simulink model "pulse_generator_V"  (R2016b)
settings: Solver=FixedStepDiscrete  StartTime=0.0  StopTime=15  RelTol=1e-3
model workspace (MAT data in the model file):
  input_struct.time = [0; 1; 2; 3; 4; 5; 6; 7; 8; 9; 10; 11; 12; 13; 14; 15; 16; 17; 18; 19; 20; 21; 22; 23; 24; 25; 26; 27; 28; 29; 30; 31; 32; 33; 34; 35; 36; 37; 38; 39; 40; 41; 42; 43; 44; 45; 46; 47; 48; 49; 50; 51; 52; 53; 54; 55; 56; 57; 58; 59; 60; 61; 62; 63; 64; 65; 66; 67; 68; 69; 70; 71; 72; 73; 74; 75; 76; 77; 78; 79; 80; 81; 82; 83; 84; 85; 86; 87; 88; 89; 90; 91; 92; 93; 94; 95; 96; 97; 98; 99; 100]
  input_struct.signals.name = 'In1'
  input_struct.signals.values = [79.4284540684; 31.1215042045; 52.8533135506; 16.56487295; 60.1981941402; 26.297128454; 65.4079098477; 68.921450314; 74.8151592824; 45.0541598502; 8.38213779969; 22.8976968717; 91.3337361502; 15.2378018969; 82.581697749; 53.834243526; 99.6134716627; 7.81755287532; 44.2678269775; 10.6652770181; 96.1898080855; 0.463422413407; 77.4910464712; 81.7303220653; 86.8694705364; 8.44358455109; 39.9782649099; 25.9870402851; 80.0068480224; 43.1413827464; 91.064759443; 18.1847028303; 26.3802916522; 14.5538980385; 13.6068558709; 86.929220764; 57.9704587366; 54.9860201836; 14.4954798224; 85.3031117722; 62.2055131485; 35.0952380892; 51.3249539867; 40.1808033752; 7.59666916908; 23.9916153554; 12.3318934835; 18.3907788282; 23.9952525665; 41.7267069084; 4.96544303257; 90.2716109915; 94.4787189722; 49.0864092468; 48.92526384; 33.7719409821; 90.0053846418; 36.924678112; 11.1202755294; 78.0252068321; 38.9738836961; 24.1691285914; 40.3912145588; 9.64545251684; 13.1973292606; 94.2050590775; 95.613454023; 57.5208595078; 5.97795429472; 23.4779913372; 35.3158571222; 82.1194040198; 1.54034376516; 4.30238016578; 16.8990029463; 64.9115474956; 73.1722385659; 64.7745963136; 45.0923706431; 54.7008892286; 29.6320805608; 74.4692807074; 18.8955015033; 68.6775433365; 18.3511155737; 36.848459649; 62.561856073; 78.0227435151; 8.11257688658; 92.9385970969; 77.5712678608; 48.6791632403; 43.5858588581; 44.678374943; 30.6349472017; 50.8508655381; 51.0771564172; 81.7627708322; 79.4831416883; 64.4318130194; 37.860938266]
  input_struct.signals.dimensions = 1
settings Model: Creator=hbourbou  LastModifiedBy=hbourbou

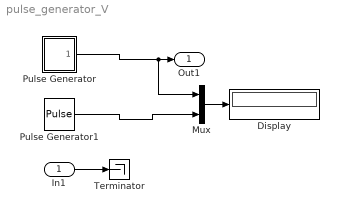
== system pulse_generator_V ==
  In1 : Inport
  Display : Display
  Mux : Mux  Inputs=2
  Pulse Generator : Subsystem  TreatAsAtomicUnit=on
  Pulse Generator1 : DiscretePulseGenerator  PulseType=Time based  Period=10  PulseWidth=5
  Terminator : Terminator
  Out1 : Outport
  wires:
  Pulse Generator/1(PG1) -> Mux/1, Out1/1
  In1/1 -> Terminator/1
  Pulse Generator1/1 -> Mux/2
  Mux/1 -> Display/1

== system pulse_generator_V/Pulse Generator ==
  PG1_gen : Subsystem  TreatAsAtomicUnit=on
  PG1 : Outport
  wires:
  PG1_gen/1(Signal) -> PG1/1

== system pulse_generator_V/Pulse Generator/PG1_gen ==
  Constant : Constant
  Sample : Gain  Gain=0.5
  Sum1 : Sum  RequirementInfo={} %GIDa_47ec9ec5_7ef4_4a83_8df2_c99b94015a05  Inputs=|++
  delay : UnitDelay  SampleTime=-1
  signal_generator : Subsystem  TreatAsAtomicUnit=on
  Signal : Outport  RequirementInfo={} %GIDa_f7ff156a_2428_4270_ba07_fd688a0637d4
  wires:
  signal_generator/1(Out) -> Signal/1
  delay/1 -> signal_generator/1(In), Sum1/2
  Constant/1 -> Sample/1
  Sum1/1 -> delay/1
  Sample/1 -> Sum1/1

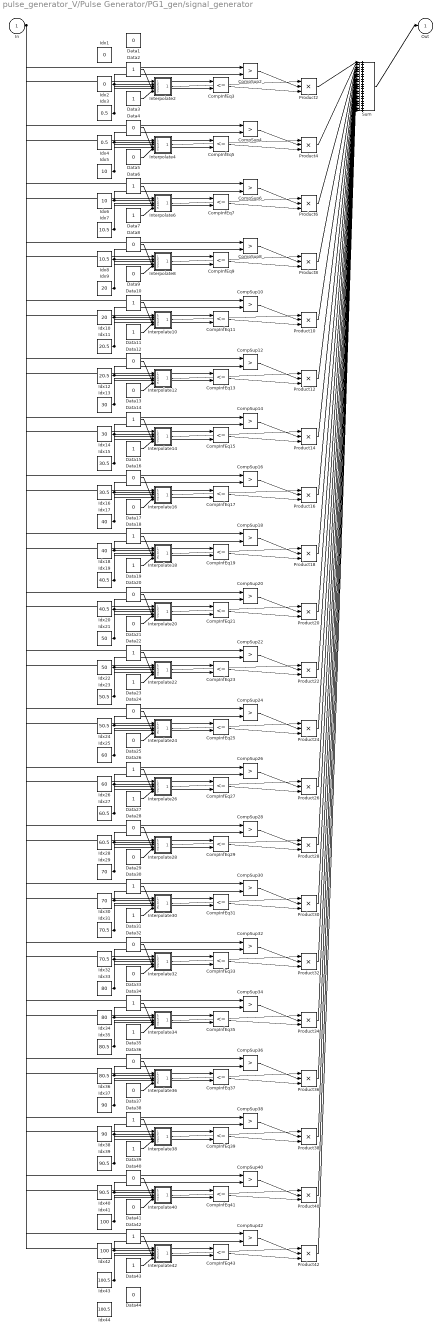
== system pulse_generator_V/Pulse Generator/PG1_gen/signal_generator ==
  In : Inport
  CompInfEq{3,5,7,9,11,13,15,17,19,21,23,25,27,29,31,33,35,37,39,41,43} (21 alike) : RelationalOperator  Operator=<=  RndMeth=Nearest  InputSameDT=on
  CompSup{2,4,6,8,10,12,14,16,18,20,22,24,26,28,30,32,34,36,38,40,42} (21 alike) : RelationalOperator  Operator=>  RndMeth=Nearest  InputSameDT=on
  Data{1,4..5,8..9,12..13,16..17,20..21,24..25,28..29,32..33,36..37,40..41,44} (22 alike) : Constant  Value=0
  Data{2..3,6..7,10..11,14..15,18..19,22..23,26..27,30..31,34..35,38..39,42..43} (22 alike) : Constant
  Idx1 : Constant  Value=0
  Idx10 : Constant  Value=20
  Idx11 : Constant  Value=20.5
  Idx12 : Constant  Value=20.5
  Idx13 : Constant  Value=30
  Idx14 : Constant  Value=30
  Idx15 : Constant  Value=30.5
  Idx16 : Constant  Value=30.5
  Idx17 : Constant  Value=40
  Idx18 : Constant  Value=40
  Idx19 : Constant  Value=40.5
  Idx2 : Constant  Value=0
  Idx20 : Constant  Value=40.5
  Idx21 : Constant  Value=50
  Idx22 : Constant  Value=50
  Idx23 : Constant  Value=50.5
  Idx24 : Constant  Value=50.5
  Idx25 : Constant  Value=60
  Idx26 : Constant  Value=60
  Idx27 : Constant  Value=60.5
  Idx28 : Constant  Value=60.5
  Idx29 : Constant  Value=70
  Idx3 : Constant  Value=0.5
  Idx30 : Constant  Value=70
  Idx31 : Constant  Value=70.5
  Idx32 : Constant  Value=70.5
  Idx33 : Constant  Value=80
  Idx34 : Constant  Value=80
  Idx35 : Constant  Value=80.5
  Idx36 : Constant  Value=80.5
  Idx37 : Constant  Value=90
  Idx38 : Constant  Value=90
  Idx39 : Constant  Value=90.5
  Idx4 : Constant  Value=0.5
  Idx40 : Constant  Value=90.5
  Idx41 : Constant  Value=100
  Idx42 : Constant  Value=100
  Idx43 : Constant  Value=100.5
  Idx44 : Constant  Value=100.5
  Idx5 : Constant  Value=10
  Idx6 : Constant  Value=10
  Idx7 : Constant  Value=10.5
  Idx8 : Constant  Value=10.5
  Idx9 : Constant  Value=20
  Interpolate10 : Subsystem  TreatAsAtomicUnit=on
  Interpolate12 : Subsystem  TreatAsAtomicUnit=on
  Interpolate14 : Subsystem  TreatAsAtomicUnit=on
  Interpolate16 : Subsystem  TreatAsAtomicUnit=on
  Interpolate18 : Subsystem  TreatAsAtomicUnit=on
  Interpolate2 : Subsystem  TreatAsAtomicUnit=on
  Interpolate20 : Subsystem  TreatAsAtomicUnit=on
  Interpolate22 : Subsystem  TreatAsAtomicUnit=on
  Interpolate24 : Subsystem  TreatAsAtomicUnit=on
  Interpolate26 : Subsystem  TreatAsAtomicUnit=on
  Interpolate28 : Subsystem  TreatAsAtomicUnit=on
  Interpolate30 : Subsystem  TreatAsAtomicUnit=on
  Interpolate32 : Subsystem  TreatAsAtomicUnit=on
  Interpolate34 : Subsystem  TreatAsAtomicUnit=on
  Interpolate36 : Subsystem  TreatAsAtomicUnit=on
  Interpolate38 : Subsystem  TreatAsAtomicUnit=on
  Interpolate4 : Subsystem  TreatAsAtomicUnit=on
  Interpolate40 : Subsystem  TreatAsAtomicUnit=on
  Interpolate42 : Subsystem  TreatAsAtomicUnit=on
  Interpolate6 : Subsystem  TreatAsAtomicUnit=on
  Interpolate8 : Subsystem  TreatAsAtomicUnit=on
  Product{2,4,6,8,10,12,14,16,18,20,22,24,26,28,30,32,34,36,38,40,42} (21 alike) : Product  Inputs=***  SaturateOnIntegerOverflow=on  RndMeth=Zero  OutDataTypeStr=Inherit: Same as first input
  Sum : Sum  Inputs=+++++++++++++++++++++  SaturateOnIntegerOverflow=on  InputSameDT=on  OutDataTypeStr=Inherit: Same as first input
  Out : Outport
  wires:
  In/1 -> Interpolate2/1(InportIn), CompSup2/1, CompInfEq3/1, Interpolate4/1(InportIn), CompSup4/1, CompInfEq5/1, Interpolate6/1(InportIn), CompSup6/1, CompInfEq7/1, Interpolate8/1(InportIn), CompSup8/1, CompInfEq9/1, Interpolate10/1(InportIn), CompSup10/1, CompInfEq11/1, Interpolate12/1(InportIn), CompSup12/1, CompInfEq13/1, Interpolate14/1(InportIn), CompSup14/1, CompInfEq15/1, Interpolate16/1(InportIn), CompSup16/1, CompInfEq17/1, Interpolate18/1(InportIn), CompSup18/1, CompInfEq19/1, Interpolate20/1(InportIn), CompSup20/1, CompInfEq21/1, Interpolate22/1(InportIn), CompSup22/1, CompInfEq23/1, Interpolate24/1(InportIn), CompSup24/1, CompInfEq25/1, Interpolate26/1(InportIn), CompSup26/1, CompInfEq27/1, Interpolate28/1(InportIn), CompSup28/1, CompInfEq29/1, Interpolate30/1(InportIn), CompSup30/1, CompInfEq31/1, Interpolate32/1(InportIn), CompSup32/1, CompInfEq33/1, Interpolate34/1(InportIn), CompSup34/1, CompInfEq35/1, Interpolate36/1(InportIn), CompSup36/1, CompInfEq37/1, Interpolate38/1(InportIn), CompSup38/1, CompInfEq39/1, Interpolate40/1(InportIn), CompSup40/1, CompInfEq41/1, Interpolate42/1(InportIn), CompSup42/1, CompInfEq43/1
  Idx2/1 -> Interpolate2/2(InportIdx1), CompSup2/2
  Data2/1 -> Interpolate2/4(InportData1)
  Interpolate2/1(Out) -> Product2/1
  CompSup2/1 -> Product2/2
  CompInfEq3/1 -> Product2/3
  Product2/1 -> Sum/1
  Idx3/1 -> Interpolate2/3(InportIdx2), CompInfEq3/2
  Data3/1 -> Interpolate2/5(InportData2)
  Idx4/1 -> Interpolate4/2(InportIdx1), CompSup4/2
  Data4/1 -> Interpolate4/4(InportData1)
  Interpolate4/1(Out) -> Product4/1
  CompSup4/1 -> Product4/2
  CompInfEq5/1 -> Product4/3
  Product4/1 -> Sum/2
  Idx5/1 -> Interpolate4/3(InportIdx2), CompInfEq5/2
  Data5/1 -> Interpolate4/5(InportData2)
  Idx6/1 -> Interpolate6/2(InportIdx1), CompSup6/2
  Data6/1 -> Interpolate6/4(InportData1)
  Interpolate6/1(Out) -> Product6/1
  CompSup6/1 -> Product6/2
  CompInfEq7/1 -> Product6/3
  Product6/1 -> Sum/3
  Idx7/1 -> Interpolate6/3(InportIdx2), CompInfEq7/2
  Data7/1 -> Interpolate6/5(InportData2)
  Idx8/1 -> Interpolate8/2(InportIdx1), CompSup8/2
  Data8/1 -> Interpolate8/4(InportData1)
  Interpolate8/1(Out) -> Product8/1
  CompSup8/1 -> Product8/2
  CompInfEq9/1 -> Product8/3
  Product8/1 -> Sum/4
  Idx9/1 -> Interpolate8/3(InportIdx2), CompInfEq9/2
  Data9/1 -> Interpolate8/5(InportData2)
  Idx10/1 -> Interpolate10/2(InportIdx1), CompSup10/2
  Data10/1 -> Interpolate10/4(InportData1)
  Interpolate10/1(Out) -> Product10/1
  CompSup10/1 -> Product10/2
  CompInfEq11/1 -> Product10/3
  Product10/1 -> Sum/5
  Idx11/1 -> Interpolate10/3(InportIdx2), CompInfEq11/2
  Data11/1 -> Interpolate10/5(InportData2)
  Idx12/1 -> Interpolate12/2(InportIdx1), CompSup12/2
  Data12/1 -> Interpolate12/4(InportData1)
  Interpolate12/1(Out) -> Product12/1
  CompSup12/1 -> Product12/2
  CompInfEq13/1 -> Product12/3
  Product12/1 -> Sum/6
  Idx13/1 -> Interpolate12/3(InportIdx2), CompInfEq13/2
  Data13/1 -> Interpolate12/5(InportData2)
  Idx14/1 -> Interpolate14/2(InportIdx1), CompSup14/2
  Data14/1 -> Interpolate14/4(InportData1)
  Interpolate14/1(Out) -> Product14/1
  CompSup14/1 -> Product14/2
  CompInfEq15/1 -> Product14/3
  Product14/1 -> Sum/7
  Idx15/1 -> Interpolate14/3(InportIdx2), CompInfEq15/2
  Data15/1 -> Interpolate14/5(InportData2)
  Idx16/1 -> Interpolate16/2(InportIdx1), CompSup16/2
  Data16/1 -> Interpolate16/4(InportData1)
  Interpolate16/1(Out) -> Product16/1
  CompSup16/1 -> Product16/2
  CompInfEq17/1 -> Product16/3
  Product16/1 -> Sum/8
  Idx17/1 -> Interpolate16/3(InportIdx2), CompInfEq17/2
  Data17/1 -> Interpolate16/5(InportData2)
  Idx18/1 -> Interpolate18/2(InportIdx1), CompSup18/2
  Data18/1 -> Interpolate18/4(InportData1)
  Interpolate18/1(Out) -> Product18/1
  CompSup18/1 -> Product18/2
  CompInfEq19/1 -> Product18/3
  Product18/1 -> Sum/9
  Idx19/1 -> Interpolate18/3(InportIdx2), CompInfEq19/2
  Data19/1 -> Interpolate18/5(InportData2)
  Idx20/1 -> Interpolate20/2(InportIdx1), CompSup20/2
  Data20/1 -> Interpolate20/4(InportData1)
  Interpolate20/1(Out) -> Product20/1
  CompSup20/1 -> Product20/2
  CompInfEq21/1 -> Product20/3
  Product20/1 -> Sum/10
  Idx21/1 -> Interpolate20/3(InportIdx2), CompInfEq21/2
  Data21/1 -> Interpolate20/5(InportData2)
  Idx22/1 -> Interpolate22/2(InportIdx1), CompSup22/2
  Data22/1 -> Interpolate22/4(InportData1)
  Interpolate22/1(Out) -> Product22/1
  CompSup22/1 -> Product22/2
  CompInfEq23/1 -> Product22/3
  Product22/1 -> Sum/11
  Idx23/1 -> Interpolate22/3(InportIdx2), CompInfEq23/2
  Data23/1 -> Interpolate22/5(InportData2)
  Idx24/1 -> Interpolate24/2(InportIdx1), CompSup24/2
  Data24/1 -> Interpolate24/4(InportData1)
  Interpolate24/1(Out) -> Product24/1
  CompSup24/1 -> Product24/2
  CompInfEq25/1 -> Product24/3
  Product24/1 -> Sum/12
  Idx25/1 -> Interpolate24/3(InportIdx2), CompInfEq25/2
  Data25/1 -> Interpolate24/5(InportData2)
  Idx26/1 -> Interpolate26/2(InportIdx1), CompSup26/2
  Data26/1 -> Interpolate26/4(InportData1)
  Interpolate26/1(Out) -> Product26/1
  CompSup26/1 -> Product26/2
  CompInfEq27/1 -> Product26/3
  Product26/1 -> Sum/13
  Idx27/1 -> Interpolate26/3(InportIdx2), CompInfEq27/2
  Data27/1 -> Interpolate26/5(InportData2)
  Idx28/1 -> Interpolate28/2(InportIdx1), CompSup28/2
  Data28/1 -> Interpolate28/4(InportData1)
  Interpolate28/1(Out) -> Product28/1
  CompSup28/1 -> Product28/2
  CompInfEq29/1 -> Product28/3
  Product28/1 -> Sum/14
  Idx29/1 -> Interpolate28/3(InportIdx2), CompInfEq29/2
  Data29/1 -> Interpolate28/5(InportData2)
  Idx30/1 -> Interpolate30/2(InportIdx1), CompSup30/2
  Data30/1 -> Interpolate30/4(InportData1)
  Interpolate30/1(Out) -> Product30/1
  CompSup30/1 -> Product30/2
  CompInfEq31/1 -> Product30/3
  Product30/1 -> Sum/15
  Idx31/1 -> Interpolate30/3(InportIdx2), CompInfEq31/2
  Data31/1 -> Interpolate30/5(InportData2)
  Idx32/1 -> Interpolate32/2(InportIdx1), CompSup32/2
  Data32/1 -> Interpolate32/4(InportData1)
  Interpolate32/1(Out) -> Product32/1
  CompSup32/1 -> Product32/2
  CompInfEq33/1 -> Product32/3
  Product32/1 -> Sum/16
  Idx33/1 -> Interpolate32/3(InportIdx2), CompInfEq33/2
  Data33/1 -> Interpolate32/5(InportData2)
  Idx34/1 -> Interpolate34/2(InportIdx1), CompSup34/2
  Data34/1 -> Interpolate34/4(InportData1)
  Interpolate34/1(Out) -> Product34/1
  CompSup34/1 -> Product34/2
  CompInfEq35/1 -> Product34/3
  Product34/1 -> Sum/17
  Idx35/1 -> Interpolate34/3(InportIdx2), CompInfEq35/2
  Data35/1 -> Interpolate34/5(InportData2)
  Idx36/1 -> Interpolate36/2(InportIdx1), CompSup36/2
  Data36/1 -> Interpolate36/4(InportData1)
  Interpolate36/1(Out) -> Product36/1
  CompSup36/1 -> Product36/2
  CompInfEq37/1 -> Product36/3
  Product36/1 -> Sum/18
  Idx37/1 -> Interpolate36/3(InportIdx2), CompInfEq37/2
  Data37/1 -> Interpolate36/5(InportData2)
  Idx38/1 -> Interpolate38/2(InportIdx1), CompSup38/2
  Data38/1 -> Interpolate38/4(InportData1)
  Interpolate38/1(Out) -> Product38/1
  CompSup38/1 -> Product38/2
  CompInfEq39/1 -> Product38/3
  Product38/1 -> Sum/19
  Idx39/1 -> Interpolate38/3(InportIdx2), CompInfEq39/2
  Data39/1 -> Interpolate38/5(InportData2)
  Idx40/1 -> Interpolate40/2(InportIdx1), CompSup40/2
  Data40/1 -> Interpolate40/4(InportData1)
  Interpolate40/1(Out) -> Product40/1
  CompSup40/1 -> Product40/2
  CompInfEq41/1 -> Product40/3
  Product40/1 -> Sum/20
  Idx41/1 -> Interpolate40/3(InportIdx2), CompInfEq41/2
  Data41/1 -> Interpolate40/5(InportData2)
  Idx42/1 -> Interpolate42/2(InportIdx1), CompSup42/2
  Data42/1 -> Interpolate42/4(InportData1)
  Interpolate42/1(Out) -> Product42/1
  CompSup42/1 -> Product42/2
  CompInfEq43/1 -> Product42/3
  Product42/1 -> Sum/21
  Idx43/1 -> Interpolate42/3(InportIdx2), CompInfEq43/2
  Data43/1 -> Interpolate42/5(InportData2)
  Sum/1 -> Out/1

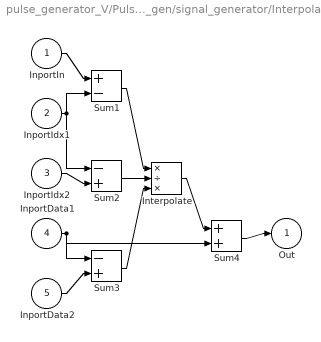
== system pulse_generator_V/Pulse Generator/PG1_gen/signal_generator/Interpolate10 ==
  InportIn : Inport
  InportIdx1 : Inport  Port=2
  InportIdx2 : Inport  Port=3
  InportData1 : Inport  Port=4
  InportData2 : Inport  Port=5
  Interpolate : Product  Inputs=*/*  SaturateOnIntegerOverflow=on  RndMeth=Zero  InputSameDT=on  OutDataTypeStr=Inherit: Same as first input
  Sum1 : Sum  Inputs=+-  SaturateOnIntegerOverflow=on  InputSameDT=on  OutDataTypeStr=Inherit: Same as first input
  Sum2 : Sum  Inputs=-+  SaturateOnIntegerOverflow=on  InputSameDT=on  OutDataTypeStr=Inherit: Same as first input
  Sum3 : Sum  Inputs=-+  SaturateOnIntegerOverflow=on  InputSameDT=on  OutDataTypeStr=Inherit: Same as first input
  Sum4 : Sum  SaturateOnIntegerOverflow=on  InputSameDT=on  OutDataTypeStr=Inherit: Same as first input
  Out : Outport
  wires:
  InportIn/1 -> Sum1/1
  InportIdx1/1 -> Sum1/2, Sum2/1
  InportIdx2/1 -> Sum2/2
  InportData1/1 -> Sum3/1, Sum4/2
  InportData2/1 -> Sum3/2
  Sum1/1 -> Interpolate/1
  Sum2/1 -> Interpolate/2
  Sum3/1 -> Interpolate/3
  Interpolate/1 -> Sum4/1
  Sum4/1 -> Out/1

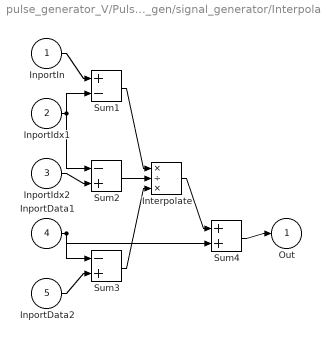
== system pulse_generator_V/Pulse Generator/PG1_gen/signal_generator/Interpolate12 ==
  InportIn : Inport
  InportIdx1 : Inport  Port=2
  InportIdx2 : Inport  Port=3
  InportData1 : Inport  Port=4
  InportData2 : Inport  Port=5
  Interpolate : Product  Inputs=*/*  SaturateOnIntegerOverflow=on  RndMeth=Zero  InputSameDT=on  OutDataTypeStr=Inherit: Same as first input
  Sum1 : Sum  Inputs=+-  SaturateOnIntegerOverflow=on  InputSameDT=on  OutDataTypeStr=Inherit: Same as first input
  Sum2 : Sum  Inputs=-+  SaturateOnIntegerOverflow=on  InputSameDT=on  OutDataTypeStr=Inherit: Same as first input
  Sum3 : Sum  Inputs=-+  SaturateOnIntegerOverflow=on  InputSameDT=on  OutDataTypeStr=Inherit: Same as first input
  Sum4 : Sum  SaturateOnIntegerOverflow=on  InputSameDT=on  OutDataTypeStr=Inherit: Same as first input
  Out : Outport
  wires:
  InportIn/1 -> Sum1/1
  InportIdx1/1 -> Sum1/2, Sum2/1
  InportIdx2/1 -> Sum2/2
  InportData1/1 -> Sum3/1, Sum4/2
  InportData2/1 -> Sum3/2
  Sum1/1 -> Interpolate/1
  Sum2/1 -> Interpolate/2
  Sum3/1 -> Interpolate/3
  Interpolate/1 -> Sum4/1
  Sum4/1 -> Out/1

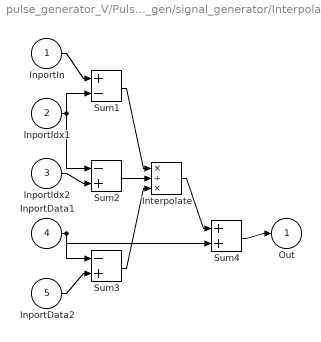
== system pulse_generator_V/Pulse Generator/PG1_gen/signal_generator/Interpolate14 ==
  InportIn : Inport
  InportIdx1 : Inport  Port=2
  InportIdx2 : Inport  Port=3
  InportData1 : Inport  Port=4
  InportData2 : Inport  Port=5
  Interpolate : Product  Inputs=*/*  SaturateOnIntegerOverflow=on  RndMeth=Zero  InputSameDT=on  OutDataTypeStr=Inherit: Same as first input
  Sum1 : Sum  Inputs=+-  SaturateOnIntegerOverflow=on  InputSameDT=on  OutDataTypeStr=Inherit: Same as first input
  Sum2 : Sum  Inputs=-+  SaturateOnIntegerOverflow=on  InputSameDT=on  OutDataTypeStr=Inherit: Same as first input
  Sum3 : Sum  Inputs=-+  SaturateOnIntegerOverflow=on  InputSameDT=on  OutDataTypeStr=Inherit: Same as first input
  Sum4 : Sum  SaturateOnIntegerOverflow=on  InputSameDT=on  OutDataTypeStr=Inherit: Same as first input
  Out : Outport
  wires:
  InportIn/1 -> Sum1/1
  InportIdx1/1 -> Sum1/2, Sum2/1
  InportIdx2/1 -> Sum2/2
  InportData1/1 -> Sum3/1, Sum4/2
  InportData2/1 -> Sum3/2
  Sum1/1 -> Interpolate/1
  Sum2/1 -> Interpolate/2
  Sum3/1 -> Interpolate/3
  Interpolate/1 -> Sum4/1
  Sum4/1 -> Out/1

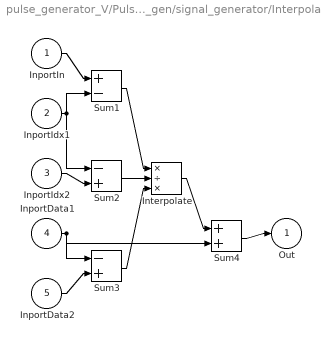
== system pulse_generator_V/Pulse Generator/PG1_gen/signal_generator/Interpolate16 ==
  InportIn : Inport
  InportIdx1 : Inport  Port=2
  InportIdx2 : Inport  Port=3
  InportData1 : Inport  Port=4
  InportData2 : Inport  Port=5
  Interpolate : Product  Inputs=*/*  SaturateOnIntegerOverflow=on  RndMeth=Zero  InputSameDT=on  OutDataTypeStr=Inherit: Same as first input
  Sum1 : Sum  Inputs=+-  SaturateOnIntegerOverflow=on  InputSameDT=on  OutDataTypeStr=Inherit: Same as first input
  Sum2 : Sum  Inputs=-+  SaturateOnIntegerOverflow=on  InputSameDT=on  OutDataTypeStr=Inherit: Same as first input
  Sum3 : Sum  Inputs=-+  SaturateOnIntegerOverflow=on  InputSameDT=on  OutDataTypeStr=Inherit: Same as first input
  Sum4 : Sum  SaturateOnIntegerOverflow=on  InputSameDT=on  OutDataTypeStr=Inherit: Same as first input
  Out : Outport
  wires:
  InportIn/1 -> Sum1/1
  InportIdx1/1 -> Sum1/2, Sum2/1
  InportIdx2/1 -> Sum2/2
  InportData1/1 -> Sum3/1, Sum4/2
  InportData2/1 -> Sum3/2
  Sum1/1 -> Interpolate/1
  Sum2/1 -> Interpolate/2
  Sum3/1 -> Interpolate/3
  Interpolate/1 -> Sum4/1
  Sum4/1 -> Out/1

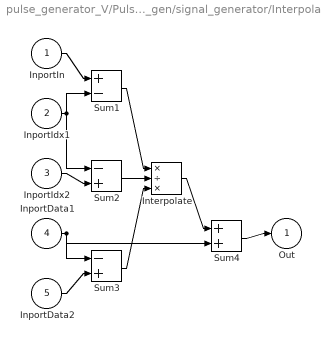
== system pulse_generator_V/Pulse Generator/PG1_gen/signal_generator/Interpolate18 ==
  InportIn : Inport
  InportIdx1 : Inport  Port=2
  InportIdx2 : Inport  Port=3
  InportData1 : Inport  Port=4
  InportData2 : Inport  Port=5
  Interpolate : Product  Inputs=*/*  SaturateOnIntegerOverflow=on  RndMeth=Zero  InputSameDT=on  OutDataTypeStr=Inherit: Same as first input
  Sum1 : Sum  Inputs=+-  SaturateOnIntegerOverflow=on  InputSameDT=on  OutDataTypeStr=Inherit: Same as first input
  Sum2 : Sum  Inputs=-+  SaturateOnIntegerOverflow=on  InputSameDT=on  OutDataTypeStr=Inherit: Same as first input
  Sum3 : Sum  Inputs=-+  SaturateOnIntegerOverflow=on  InputSameDT=on  OutDataTypeStr=Inherit: Same as first input
  Sum4 : Sum  SaturateOnIntegerOverflow=on  InputSameDT=on  OutDataTypeStr=Inherit: Same as first input
  Out : Outport
  wires:
  InportIn/1 -> Sum1/1
  InportIdx1/1 -> Sum1/2, Sum2/1
  InportIdx2/1 -> Sum2/2
  InportData1/1 -> Sum3/1, Sum4/2
  InportData2/1 -> Sum3/2
  Sum1/1 -> Interpolate/1
  Sum2/1 -> Interpolate/2
  Sum3/1 -> Interpolate/3
  Interpolate/1 -> Sum4/1
  Sum4/1 -> Out/1

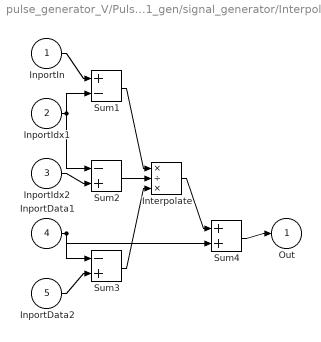
== system pulse_generator_V/Pulse Generator/PG1_gen/signal_generator/Interpolate2 ==
  InportIn : Inport
  InportIdx1 : Inport  Port=2
  InportIdx2 : Inport  Port=3
  InportData1 : Inport  Port=4
  InportData2 : Inport  Port=5
  Interpolate : Product  Inputs=*/*  SaturateOnIntegerOverflow=on  RndMeth=Zero  InputSameDT=on  OutDataTypeStr=Inherit: Same as first input
  Sum1 : Sum  Inputs=+-  SaturateOnIntegerOverflow=on  InputSameDT=on  OutDataTypeStr=Inherit: Same as first input
  Sum2 : Sum  Inputs=-+  SaturateOnIntegerOverflow=on  InputSameDT=on  OutDataTypeStr=Inherit: Same as first input
  Sum3 : Sum  Inputs=-+  SaturateOnIntegerOverflow=on  InputSameDT=on  OutDataTypeStr=Inherit: Same as first input
  Sum4 : Sum  SaturateOnIntegerOverflow=on  InputSameDT=on  OutDataTypeStr=Inherit: Same as first input
  Out : Outport
  wires:
  InportIn/1 -> Sum1/1
  InportIdx1/1 -> Sum1/2, Sum2/1
  InportIdx2/1 -> Sum2/2
  InportData1/1 -> Sum3/1, Sum4/2
  InportData2/1 -> Sum3/2
  Sum1/1 -> Interpolate/1
  Sum2/1 -> Interpolate/2
  Sum3/1 -> Interpolate/3
  Interpolate/1 -> Sum4/1
  Sum4/1 -> Out/1

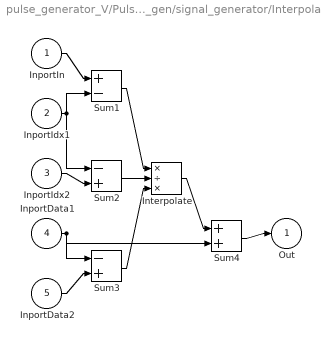
== system pulse_generator_V/Pulse Generator/PG1_gen/signal_generator/Interpolate20 ==
  InportIn : Inport
  InportIdx1 : Inport  Port=2
  InportIdx2 : Inport  Port=3
  InportData1 : Inport  Port=4
  InportData2 : Inport  Port=5
  Interpolate : Product  Inputs=*/*  SaturateOnIntegerOverflow=on  RndMeth=Zero  InputSameDT=on  OutDataTypeStr=Inherit: Same as first input
  Sum1 : Sum  Inputs=+-  SaturateOnIntegerOverflow=on  InputSameDT=on  OutDataTypeStr=Inherit: Same as first input
  Sum2 : Sum  Inputs=-+  SaturateOnIntegerOverflow=on  InputSameDT=on  OutDataTypeStr=Inherit: Same as first input
  Sum3 : Sum  Inputs=-+  SaturateOnIntegerOverflow=on  InputSameDT=on  OutDataTypeStr=Inherit: Same as first input
  Sum4 : Sum  SaturateOnIntegerOverflow=on  InputSameDT=on  OutDataTypeStr=Inherit: Same as first input
  Out : Outport
  wires:
  InportIn/1 -> Sum1/1
  InportIdx1/1 -> Sum1/2, Sum2/1
  InportIdx2/1 -> Sum2/2
  InportData1/1 -> Sum3/1, Sum4/2
  InportData2/1 -> Sum3/2
  Sum1/1 -> Interpolate/1
  Sum2/1 -> Interpolate/2
  Sum3/1 -> Interpolate/3
  Interpolate/1 -> Sum4/1
  Sum4/1 -> Out/1

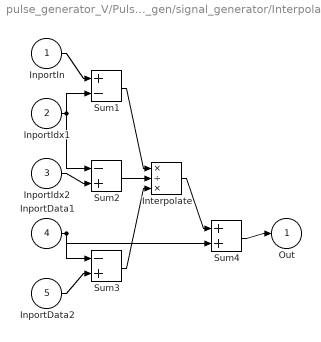
== system pulse_generator_V/Pulse Generator/PG1_gen/signal_generator/Interpolate22 ==
  InportIn : Inport
  InportIdx1 : Inport  Port=2
  InportIdx2 : Inport  Port=3
  InportData1 : Inport  Port=4
  InportData2 : Inport  Port=5
  Interpolate : Product  Inputs=*/*  SaturateOnIntegerOverflow=on  RndMeth=Zero  InputSameDT=on  OutDataTypeStr=Inherit: Same as first input
  Sum1 : Sum  Inputs=+-  SaturateOnIntegerOverflow=on  InputSameDT=on  OutDataTypeStr=Inherit: Same as first input
  Sum2 : Sum  Inputs=-+  SaturateOnIntegerOverflow=on  InputSameDT=on  OutDataTypeStr=Inherit: Same as first input
  Sum3 : Sum  Inputs=-+  SaturateOnIntegerOverflow=on  InputSameDT=on  OutDataTypeStr=Inherit: Same as first input
  Sum4 : Sum  SaturateOnIntegerOverflow=on  InputSameDT=on  OutDataTypeStr=Inherit: Same as first input
  Out : Outport
  wires:
  InportIn/1 -> Sum1/1
  InportIdx1/1 -> Sum1/2, Sum2/1
  InportIdx2/1 -> Sum2/2
  InportData1/1 -> Sum3/1, Sum4/2
  InportData2/1 -> Sum3/2
  Sum1/1 -> Interpolate/1
  Sum2/1 -> Interpolate/2
  Sum3/1 -> Interpolate/3
  Interpolate/1 -> Sum4/1
  Sum4/1 -> Out/1

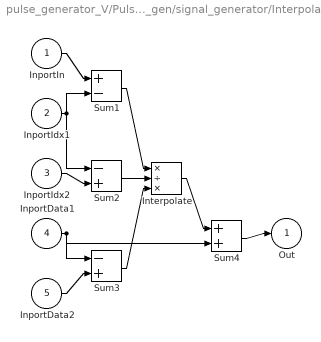
== system pulse_generator_V/Pulse Generator/PG1_gen/signal_generator/Interpolate24 ==
  InportIn : Inport
  InportIdx1 : Inport  Port=2
  InportIdx2 : Inport  Port=3
  InportData1 : Inport  Port=4
  InportData2 : Inport  Port=5
  Interpolate : Product  Inputs=*/*  SaturateOnIntegerOverflow=on  RndMeth=Zero  InputSameDT=on  OutDataTypeStr=Inherit: Same as first input
  Sum1 : Sum  Inputs=+-  SaturateOnIntegerOverflow=on  InputSameDT=on  OutDataTypeStr=Inherit: Same as first input
  Sum2 : Sum  Inputs=-+  SaturateOnIntegerOverflow=on  InputSameDT=on  OutDataTypeStr=Inherit: Same as first input
  Sum3 : Sum  Inputs=-+  SaturateOnIntegerOverflow=on  InputSameDT=on  OutDataTypeStr=Inherit: Same as first input
  Sum4 : Sum  SaturateOnIntegerOverflow=on  InputSameDT=on  OutDataTypeStr=Inherit: Same as first input
  Out : Outport
  wires:
  InportIn/1 -> Sum1/1
  InportIdx1/1 -> Sum1/2, Sum2/1
  InportIdx2/1 -> Sum2/2
  InportData1/1 -> Sum3/1, Sum4/2
  InportData2/1 -> Sum3/2
  Sum1/1 -> Interpolate/1
  Sum2/1 -> Interpolate/2
  Sum3/1 -> Interpolate/3
  Interpolate/1 -> Sum4/1
  Sum4/1 -> Out/1

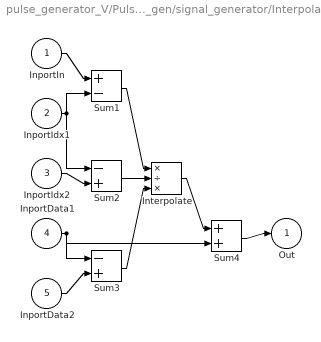
== system pulse_generator_V/Pulse Generator/PG1_gen/signal_generator/Interpolate26 ==
  InportIn : Inport
  InportIdx1 : Inport  Port=2
  InportIdx2 : Inport  Port=3
  InportData1 : Inport  Port=4
  InportData2 : Inport  Port=5
  Interpolate : Product  Inputs=*/*  SaturateOnIntegerOverflow=on  RndMeth=Zero  InputSameDT=on  OutDataTypeStr=Inherit: Same as first input
  Sum1 : Sum  Inputs=+-  SaturateOnIntegerOverflow=on  InputSameDT=on  OutDataTypeStr=Inherit: Same as first input
  Sum2 : Sum  Inputs=-+  SaturateOnIntegerOverflow=on  InputSameDT=on  OutDataTypeStr=Inherit: Same as first input
  Sum3 : Sum  Inputs=-+  SaturateOnIntegerOverflow=on  InputSameDT=on  OutDataTypeStr=Inherit: Same as first input
  Sum4 : Sum  SaturateOnIntegerOverflow=on  InputSameDT=on  OutDataTypeStr=Inherit: Same as first input
  Out : Outport
  wires:
  InportIn/1 -> Sum1/1
  InportIdx1/1 -> Sum1/2, Sum2/1
  InportIdx2/1 -> Sum2/2
  InportData1/1 -> Sum3/1, Sum4/2
  InportData2/1 -> Sum3/2
  Sum1/1 -> Interpolate/1
  Sum2/1 -> Interpolate/2
  Sum3/1 -> Interpolate/3
  Interpolate/1 -> Sum4/1
  Sum4/1 -> Out/1

== system pulse_generator_V/Pulse Generator/PG1_gen/signal_generator/Interpolate28 ==
  InportIn : Inport
  InportIdx1 : Inport  Port=2
  InportIdx2 : Inport  Port=3
  InportData1 : Inport  Port=4
  InportData2 : Inport  Port=5
  Interpolate : Product  Inputs=*/*  SaturateOnIntegerOverflow=on  RndMeth=Zero  InputSameDT=on  OutDataTypeStr=Inherit: Same as first input
  Sum1 : Sum  Inputs=+-  SaturateOnIntegerOverflow=on  InputSameDT=on  OutDataTypeStr=Inherit: Same as first input
  Sum2 : Sum  Inputs=-+  SaturateOnIntegerOverflow=on  InputSameDT=on  OutDataTypeStr=Inherit: Same as first input
  Sum3 : Sum  Inputs=-+  SaturateOnIntegerOverflow=on  InputSameDT=on  OutDataTypeStr=Inherit: Same as first input
  Sum4 : Sum  SaturateOnIntegerOverflow=on  InputSameDT=on  OutDataTypeStr=Inherit: Same as first input
  Out : Outport
  wires:
  InportIn/1 -> Sum1/1
  InportIdx1/1 -> Sum1/2, Sum2/1
  InportIdx2/1 -> Sum2/2
  InportData1/1 -> Sum3/1, Sum4/2
  InportData2/1 -> Sum3/2
  Sum1/1 -> Interpolate/1
  Sum2/1 -> Interpolate/2
  Sum3/1 -> Interpolate/3
  Interpolate/1 -> Sum4/1
  Sum4/1 -> Out/1

== system pulse_generator_V/Pulse Generator/PG1_gen/signal_generator/Interpolate30 ==
  InportIn : Inport
  InportIdx1 : Inport  Port=2
  InportIdx2 : Inport  Port=3
  InportData1 : Inport  Port=4
  InportData2 : Inport  Port=5
  Interpolate : Product  Inputs=*/*  SaturateOnIntegerOverflow=on  RndMeth=Zero  InputSameDT=on  OutDataTypeStr=Inherit: Same as first input
  Sum1 : Sum  Inputs=+-  SaturateOnIntegerOverflow=on  InputSameDT=on  OutDataTypeStr=Inherit: Same as first input
  Sum2 : Sum  Inputs=-+  SaturateOnIntegerOverflow=on  InputSameDT=on  OutDataTypeStr=Inherit: Same as first input
  Sum3 : Sum  Inputs=-+  SaturateOnIntegerOverflow=on  InputSameDT=on  OutDataTypeStr=Inherit: Same as first input
  Sum4 : Sum  SaturateOnIntegerOverflow=on  InputSameDT=on  OutDataTypeStr=Inherit: Same as first input
  Out : Outport
  wires:
  InportIn/1 -> Sum1/1
  InportIdx1/1 -> Sum1/2, Sum2/1
  InportIdx2/1 -> Sum2/2
  InportData1/1 -> Sum3/1, Sum4/2
  InportData2/1 -> Sum3/2
  Sum1/1 -> Interpolate/1
  Sum2/1 -> Interpolate/2
  Sum3/1 -> Interpolate/3
  Interpolate/1 -> Sum4/1
  Sum4/1 -> Out/1

== system pulse_generator_V/Pulse Generator/PG1_gen/signal_generator/Interpolate32 ==
  InportIn : Inport
  InportIdx1 : Inport  Port=2
  InportIdx2 : Inport  Port=3
  InportData1 : Inport  Port=4
  InportData2 : Inport  Port=5
  Interpolate : Product  Inputs=*/*  SaturateOnIntegerOverflow=on  RndMeth=Zero  InputSameDT=on  OutDataTypeStr=Inherit: Same as first input
  Sum1 : Sum  Inputs=+-  SaturateOnIntegerOverflow=on  InputSameDT=on  OutDataTypeStr=Inherit: Same as first input
  Sum2 : Sum  Inputs=-+  SaturateOnIntegerOverflow=on  InputSameDT=on  OutDataTypeStr=Inherit: Same as first input
  Sum3 : Sum  Inputs=-+  SaturateOnIntegerOverflow=on  InputSameDT=on  OutDataTypeStr=Inherit: Same as first input
  Sum4 : Sum  SaturateOnIntegerOverflow=on  InputSameDT=on  OutDataTypeStr=Inherit: Same as first input
  Out : Outport
  wires:
  InportIn/1 -> Sum1/1
  InportIdx1/1 -> Sum1/2, Sum2/1
  InportIdx2/1 -> Sum2/2
  InportData1/1 -> Sum3/1, Sum4/2
  InportData2/1 -> Sum3/2
  Sum1/1 -> Interpolate/1
  Sum2/1 -> Interpolate/2
  Sum3/1 -> Interpolate/3
  Interpolate/1 -> Sum4/1
  Sum4/1 -> Out/1

== system pulse_generator_V/Pulse Generator/PG1_gen/signal_generator/Interpolate34 ==
  InportIn : Inport
  InportIdx1 : Inport  Port=2
  InportIdx2 : Inport  Port=3
  InportData1 : Inport  Port=4
  InportData2 : Inport  Port=5
  Interpolate : Product  Inputs=*/*  SaturateOnIntegerOverflow=on  RndMeth=Zero  InputSameDT=on  OutDataTypeStr=Inherit: Same as first input
  Sum1 : Sum  Inputs=+-  SaturateOnIntegerOverflow=on  InputSameDT=on  OutDataTypeStr=Inherit: Same as first input
  Sum2 : Sum  Inputs=-+  SaturateOnIntegerOverflow=on  InputSameDT=on  OutDataTypeStr=Inherit: Same as first input
  Sum3 : Sum  Inputs=-+  SaturateOnIntegerOverflow=on  InputSameDT=on  OutDataTypeStr=Inherit: Same as first input
  Sum4 : Sum  SaturateOnIntegerOverflow=on  InputSameDT=on  OutDataTypeStr=Inherit: Same as first input
  Out : Outport
  wires:
  InportIn/1 -> Sum1/1
  InportIdx1/1 -> Sum1/2, Sum2/1
  InportIdx2/1 -> Sum2/2
  InportData1/1 -> Sum3/1, Sum4/2
  InportData2/1 -> Sum3/2
  Sum1/1 -> Interpolate/1
  Sum2/1 -> Interpolate/2
  Sum3/1 -> Interpolate/3
  Interpolate/1 -> Sum4/1
  Sum4/1 -> Out/1

== system pulse_generator_V/Pulse Generator/PG1_gen/signal_generator/Interpolate36 ==
  InportIn : Inport
  InportIdx1 : Inport  Port=2
  InportIdx2 : Inport  Port=3
  InportData1 : Inport  Port=4
  InportData2 : Inport  Port=5
  Interpolate : Product  Inputs=*/*  SaturateOnIntegerOverflow=on  RndMeth=Zero  InputSameDT=on  OutDataTypeStr=Inherit: Same as first input
  Sum1 : Sum  Inputs=+-  SaturateOnIntegerOverflow=on  InputSameDT=on  OutDataTypeStr=Inherit: Same as first input
  Sum2 : Sum  Inputs=-+  SaturateOnIntegerOverflow=on  InputSameDT=on  OutDataTypeStr=Inherit: Same as first input
  Sum3 : Sum  Inputs=-+  SaturateOnIntegerOverflow=on  InputSameDT=on  OutDataTypeStr=Inherit: Same as first input
  Sum4 : Sum  SaturateOnIntegerOverflow=on  InputSameDT=on  OutDataTypeStr=Inherit: Same as first input
  Out : Outport
  wires:
  InportIn/1 -> Sum1/1
  InportIdx1/1 -> Sum1/2, Sum2/1
  InportIdx2/1 -> Sum2/2
  InportData1/1 -> Sum3/1, Sum4/2
  InportData2/1 -> Sum3/2
  Sum1/1 -> Interpolate/1
  Sum2/1 -> Interpolate/2
  Sum3/1 -> Interpolate/3
  Interpolate/1 -> Sum4/1
  Sum4/1 -> Out/1

== system pulse_generator_V/Pulse Generator/PG1_gen/signal_generator/Interpolate38 ==
  InportIn : Inport
  InportIdx1 : Inport  Port=2
  InportIdx2 : Inport  Port=3
  InportData1 : Inport  Port=4
  InportData2 : Inport  Port=5
  Interpolate : Product  Inputs=*/*  SaturateOnIntegerOverflow=on  RndMeth=Zero  InputSameDT=on  OutDataTypeStr=Inherit: Same as first input
  Sum1 : Sum  Inputs=+-  SaturateOnIntegerOverflow=on  InputSameDT=on  OutDataTypeStr=Inherit: Same as first input
  Sum2 : Sum  Inputs=-+  SaturateOnIntegerOverflow=on  InputSameDT=on  OutDataTypeStr=Inherit: Same as first input
  Sum3 : Sum  Inputs=-+  SaturateOnIntegerOverflow=on  InputSameDT=on  OutDataTypeStr=Inherit: Same as first input
  Sum4 : Sum  SaturateOnIntegerOverflow=on  InputSameDT=on  OutDataTypeStr=Inherit: Same as first input
  Out : Outport
  wires:
  InportIn/1 -> Sum1/1
  InportIdx1/1 -> Sum1/2, Sum2/1
  InportIdx2/1 -> Sum2/2
  InportData1/1 -> Sum3/1, Sum4/2
  InportData2/1 -> Sum3/2
  Sum1/1 -> Interpolate/1
  Sum2/1 -> Interpolate/2
  Sum3/1 -> Interpolate/3
  Interpolate/1 -> Sum4/1
  Sum4/1 -> Out/1

== system pulse_generator_V/Pulse Generator/PG1_gen/signal_generator/Interpolate4 ==
  InportIn : Inport
  InportIdx1 : Inport  Port=2
  InportIdx2 : Inport  Port=3
  InportData1 : Inport  Port=4
  InportData2 : Inport  Port=5
  Interpolate : Product  Inputs=*/*  SaturateOnIntegerOverflow=on  RndMeth=Zero  InputSameDT=on  OutDataTypeStr=Inherit: Same as first input
  Sum1 : Sum  Inputs=+-  SaturateOnIntegerOverflow=on  InputSameDT=on  OutDataTypeStr=Inherit: Same as first input
  Sum2 : Sum  Inputs=-+  SaturateOnIntegerOverflow=on  InputSameDT=on  OutDataTypeStr=Inherit: Same as first input
  Sum3 : Sum  Inputs=-+  SaturateOnIntegerOverflow=on  InputSameDT=on  OutDataTypeStr=Inherit: Same as first input
  Sum4 : Sum  SaturateOnIntegerOverflow=on  InputSameDT=on  OutDataTypeStr=Inherit: Same as first input
  Out : Outport
  wires:
  InportIn/1 -> Sum1/1
  InportIdx1/1 -> Sum1/2, Sum2/1
  InportIdx2/1 -> Sum2/2
  InportData1/1 -> Sum3/1, Sum4/2
  InportData2/1 -> Sum3/2
  Sum1/1 -> Interpolate/1
  Sum2/1 -> Interpolate/2
  Sum3/1 -> Interpolate/3
  Interpolate/1 -> Sum4/1
  Sum4/1 -> Out/1

== system pulse_generator_V/Pulse Generator/PG1_gen/signal_generator/Interpolate40 ==
  InportIn : Inport
  InportIdx1 : Inport  Port=2
  InportIdx2 : Inport  Port=3
  InportData1 : Inport  Port=4
  InportData2 : Inport  Port=5
  Interpolate : Product  Inputs=*/*  SaturateOnIntegerOverflow=on  RndMeth=Zero  InputSameDT=on  OutDataTypeStr=Inherit: Same as first input
  Sum1 : Sum  Inputs=+-  SaturateOnIntegerOverflow=on  InputSameDT=on  OutDataTypeStr=Inherit: Same as first input
  Sum2 : Sum  Inputs=-+  SaturateOnIntegerOverflow=on  InputSameDT=on  OutDataTypeStr=Inherit: Same as first input
  Sum3 : Sum  Inputs=-+  SaturateOnIntegerOverflow=on  InputSameDT=on  OutDataTypeStr=Inherit: Same as first input
  Sum4 : Sum  SaturateOnIntegerOverflow=on  InputSameDT=on  OutDataTypeStr=Inherit: Same as first input
  Out : Outport
  wires:
  InportIn/1 -> Sum1/1
  InportIdx1/1 -> Sum1/2, Sum2/1
  InportIdx2/1 -> Sum2/2
  InportData1/1 -> Sum3/1, Sum4/2
  InportData2/1 -> Sum3/2
  Sum1/1 -> Interpolate/1
  Sum2/1 -> Interpolate/2
  Sum3/1 -> Interpolate/3
  Interpolate/1 -> Sum4/1
  Sum4/1 -> Out/1

== system pulse_generator_V/Pulse Generator/PG1_gen/signal_generator/Interpolate42 ==
  InportIn : Inport
  InportIdx1 : Inport  Port=2
  InportIdx2 : Inport  Port=3
  InportData1 : Inport  Port=4
  InportData2 : Inport  Port=5
  Interpolate : Product  Inputs=*/*  SaturateOnIntegerOverflow=on  RndMeth=Zero  InputSameDT=on  OutDataTypeStr=Inherit: Same as first input
  Sum1 : Sum  Inputs=+-  SaturateOnIntegerOverflow=on  InputSameDT=on  OutDataTypeStr=Inherit: Same as first input
  Sum2 : Sum  Inputs=-+  SaturateOnIntegerOverflow=on  InputSameDT=on  OutDataTypeStr=Inherit: Same as first input
  Sum3 : Sum  Inputs=-+  SaturateOnIntegerOverflow=on  InputSameDT=on  OutDataTypeStr=Inherit: Same as first input
  Sum4 : Sum  SaturateOnIntegerOverflow=on  InputSameDT=on  OutDataTypeStr=Inherit: Same as first input
  Out : Outport
  wires:
  InportIn/1 -> Sum1/1
  InportIdx1/1 -> Sum1/2, Sum2/1
  InportIdx2/1 -> Sum2/2
  InportData1/1 -> Sum3/1, Sum4/2
  InportData2/1 -> Sum3/2
  Sum1/1 -> Interpolate/1
  Sum2/1 -> Interpolate/2
  Sum3/1 -> Interpolate/3
  Interpolate/1 -> Sum4/1
  Sum4/1 -> Out/1

== system pulse_generator_V/Pulse Generator/PG1_gen/signal_generator/Interpolate6 ==
  InportIn : Inport
  InportIdx1 : Inport  Port=2
  InportIdx2 : Inport  Port=3
  InportData1 : Inport  Port=4
  InportData2 : Inport  Port=5
  Interpolate : Product  Inputs=*/*  SaturateOnIntegerOverflow=on  RndMeth=Zero  InputSameDT=on  OutDataTypeStr=Inherit: Same as first input
  Sum1 : Sum  Inputs=+-  SaturateOnIntegerOverflow=on  InputSameDT=on  OutDataTypeStr=Inherit: Same as first input
  Sum2 : Sum  Inputs=-+  SaturateOnIntegerOverflow=on  InputSameDT=on  OutDataTypeStr=Inherit: Same as first input
  Sum3 : Sum  Inputs=-+  SaturateOnIntegerOverflow=on  InputSameDT=on  OutDataTypeStr=Inherit: Same as first input
  Sum4 : Sum  SaturateOnIntegerOverflow=on  InputSameDT=on  OutDataTypeStr=Inherit: Same as first input
  Out : Outport
  wires:
  InportIn/1 -> Sum1/1
  InportIdx1/1 -> Sum1/2, Sum2/1
  InportIdx2/1 -> Sum2/2
  InportData1/1 -> Sum3/1, Sum4/2
  InportData2/1 -> Sum3/2
  Sum1/1 -> Interpolate/1
  Sum2/1 -> Interpolate/2
  Sum3/1 -> Interpolate/3
  Interpolate/1 -> Sum4/1
  Sum4/1 -> Out/1

== system pulse_generator_V/Pulse Generator/PG1_gen/signal_generator/Interpolate8 ==
  InportIn : Inport
  InportIdx1 : Inport  Port=2
  InportIdx2 : Inport  Port=3
  InportData1 : Inport  Port=4
  InportData2 : Inport  Port=5
  Interpolate : Product  Inputs=*/*  SaturateOnIntegerOverflow=on  RndMeth=Zero  InputSameDT=on  OutDataTypeStr=Inherit: Same as first input
  Sum1 : Sum  Inputs=+-  SaturateOnIntegerOverflow=on  InputSameDT=on  OutDataTypeStr=Inherit: Same as first input
  Sum2 : Sum  Inputs=-+  SaturateOnIntegerOverflow=on  InputSameDT=on  OutDataTypeStr=Inherit: Same as first input
  Sum3 : Sum  Inputs=-+  SaturateOnIntegerOverflow=on  InputSameDT=on  OutDataTypeStr=Inherit: Same as first input
  Sum4 : Sum  SaturateOnIntegerOverflow=on  InputSameDT=on  OutDataTypeStr=Inherit: Same as first input
  Out : Outport
  wires:
  InportIn/1 -> Sum1/1
  InportIdx1/1 -> Sum1/2, Sum2/1
  InportIdx2/1 -> Sum2/2
  InportData1/1 -> Sum3/1, Sum4/2
  InportData2/1 -> Sum3/2
  Sum1/1 -> Interpolate/1
  Sum2/1 -> Interpolate/2
  Sum3/1 -> Interpolate/3
  Interpolate/1 -> Sum4/1
  Sum4/1 -> Out/1
